simulink model "BuckyWagon_01"  (Simulink 7.7)
settings: Solver=FixedStepDiscrete  StartTime=0.0  StopTime=10.0  RelTol=1e-3
PreLoadFcn:
  | try, eval([bdroot '_setup']); catch, eval('model_setup', ''); end
InitFcn:
  | try, eval([bdroot '_setup']); catch, eval('model_setup', ''); end
undefined symbols (not defined in the file or in its folder): ECU565, High, Low, miniviewSetup, motohawk_build_version, motohawk_get_faults, motohawk_setup_toolchains, motohawk_trunc_name, motohawk_vardec_config_group, motohawk_vardec_path, tc, True
libraries: MotoHawk_lib x594, simulink x27, motohawk_control_primitives_lib x19, miniview_lib x10, MotoHawk_VDOGauge_lib x8, motohawk_engine_lib x5, motohawk_annotations_lib x1
(part 5 of 10)

== system BuckyWagon_01/Foreground/Control Strategy/HV Controller ==
  Battery Ready : Inport
  Contactor Status : Inport  Port=2
  Eaton  Present : Inport  Port=3
  Drive Ready : Inport  Port=4
  Charge Contactor : Inport  Port=5
  Battery has passed power-on-self-test and is ready : simulink/Logic and Bit Operations/Compare To Constant  SystemSampleTime=-1  relop===  const=1  LogicOutDataTypeMode=boolean
  Contacter Controller : Subsystem
  Logical Operator{,1,3..4} (4 alike) : Logic  AllPortsSameDT=off  OutDataTypeStr=boolean
  Logical Operator12 : Logic  Operator=OR  AllPortsSameDT=off  OutDataTypeStr=boolean
  Logical Operator2 : Logic  Operator=NOT  AllPortsSameDT=off  OutDataTypeStr=boolean
  Logical Operator5 : Logic  Operator=OR  AllPortsSameDT=off  OutDataTypeStr=boolean
  Main contactors closed and ready : simulink/Logic and Bit Operations/Compare To Constant  SystemSampleTime=-1  relop===  const=1  LogicOutDataTypeMode=boolean
  motohawk_calibration8 : MotoHawk_lib/Calibration & Probing Blocks/motohawk_calibration  nam='Allow_MainContactor_Close'  val=16  storage=Calibration  show_more=on  name_source=Use Parameter  data_type=boolean  read_level=1  write_level=1  ovr_cals=on  view_as=Number  enum_struct={'Disabled', 'Enabled'}  vector_style=Wide Row  use_help_units=on  help='1=normal mode, 0=prevent main contactors from closing'  units='flag'  use_header_enum=off  row_header_enum={}  col_header_enum={}  use_min_max=on  min_val=0  max_val=1  use_precision=off  precision=''  gain=1  offset=0  exp=1  use_mototune_group=on  mototune_group='Actuators | BCM'
  motohawk_data_def2 : MotoHawk_lib/Data Storage Blocks/motohawk_data_def  nam='Batt_Load_Enable'  container_nam=''  data=0  typ=boolean  struct_nam='MyStruct'  storage=Volatile  outputRef=off  use_vardec=on  window=Display  read_level=1  write_level=1  ovr_cals=on  view_as=Number  enum_struct={'Disabled', 'Enabled'}  vector_style=Wide Row  use_help_units=off  help=''  units=''  use_header_enum=off  row_header_enum=''  col_header_enum=''  use_min_max=off  min_val=-inf  max_val=inf  use_precision=off  precision=''  gain=1  offset=0  exp=1  use_mototune_group=off  mototune_group=motohawk_vardec_path(gcb)  eval_name=MyData  data_stores=motohawk_sfun_data_def_data_stores  struct_instances=motohawk_sfun_data_def_struct_instances  vardecs=motohawk_sfun_data_def_vardecs
  motohawk_data_read : MotoHawk_lib/Data Storage Blocks/motohawk_data_read  source=Lookup By Name  structure=Scalar  operation=Read scalar from location by index  sz_vec=4  sz_row=2  sz_col=3  typ=boolean  nam='Shutdown_Req'  checkNull=on  struct_inst_name='Struct1'  struct_nam='MyStruct'
  motohawk_data_write : MotoHawk_lib/Data Storage Blocks/motohawk_data_write  source=Lookup By Name  structure=Scalar  operation=Write entire data structure at once  sz_vec=9  sz_row=2  sz_col=9  typ=boolean  nam='Batt_Load_Enable'  checkNull=on  write_read_only=off  struct_inst_name=''  struct_name='MyStruct'
  motohawk_fault_action : MotoHawk_lib/Fault Management Blocks/motohawk_fault_action  nam='OpenContactors'  output_status=on  eval_nam=OpenContactors
  motohawk_override_abs2 : MotoHawk_lib/Calibration & Probing Blocks/motohawk_override_abs  SystemSampleTime=-1  parent_name='Contactor_Shutdown_Test'  parent_val=0  show_more=on  name_source=Use Parameter  parent_read_level=1  parent_override_level=1  view_as=Number  enum_struct={'Disabled', 'Enabled'}  use_help_units=off  parent_help=''  parent_units=''  use_min_max=on  parent_min=0  parent_max=1  use_precision=off  parent_precision=''  parent_gain=1  parent_offset=0  parent_exp=1  use_mototune_group=on  parent_group='BuckyWagon_01 | Strategy | Control Strategy | HV Controller'
  Contactor Command : Outport
  DC DC Enable : Outport  Port=2
  Drive Enable : Outport  Port=3
  HV Hydraulic Pump Enable : Outport  Port=4
  wires:
  Battery Ready/1 -> Battery has passed power-on-self-test and is ready/1
  Contactor Status/1 -> Main contactors closed and ready/1
  Battery has passed power-on-self-test and is ready/1 -> Contacter Controller/1(Battery OK)
  Main contactors closed and ready/1 -> Contacter Controller/3(Contactor Status)
  Contacter Controller/1(Contactor Enable) -> Logical Operator/2
  Logical Operator/1 -> Contactor Command/1
  motohawk_calibration8/1 -> Logical Operator/1
  Logical Operator12/1 -> Contacter Controller/2(Shutdown Command)
  motohawk_override_abs2/1 -> Logical Operator12/1
  motohawk_fault_action/1 -> Logical Operator12/2
  Eaton  Present/1 -> Logical Operator2/1
  motohawk_data_read/1 -> Logical Operator1/1
  Logical Operator1/1 -> motohawk_override_abs2/1
  Logical Operator2/1 -> Logical Operator1/2, Logical Operator3/2
  Contacter Controller/2(Load Enable) -> Logical Operator3/1, motohawk_data_write/1, Logical Operator5/1
  Logical Operator3/1 -> Logical Operator4/2, HV Hydraulic Pump Enable/1
  Logical Operator4/1 -> Drive Enable/1
  Drive Ready/1 -> Logical Operator4/1
  Logical Operator5/1 -> DC DC Enable/1
  Charge Contactor/1 -> Logical Operator5/2

== system BuckyWagon_01/Foreground/Control Strategy/Reverse ==
  Inputs : Inport
  Abs : Abs
  Bus Selector2 : BusSelector  OutputSignals=Accel,VehicleSpeed,ReverseSw
  Chart : Stateflow chart  TreatAsAtomicUnit=on
  Constant : Constant
  Switch : Switch  Criteria=u2 ~= 0
  motohawk_calibration : MotoHawk_lib/Calibration & Probing Blocks/motohawk_calibration  nam='fwdAccThres'  val=0.02  storage=Calibration  show_more=on  name_source=Use Parameter  data_type=Inherit from 'Default Value'  read_level=1  write_level=1  ovr_cals=on  view_as=Number  enum_struct={'Disabled', 'Enabled'}  vector_style=Wide Row  use_help_units=on  help='Accelerator must be below this to switch Rev->Fwd'  units='%'  use_header_enum=off  row_header_enum={}  col_header_enum={}  use_min_max=on  min_val=0  max_val=1  use_precision=off  precision=''  gain=1  offset=0  exp=1  use_mototune_group=off  mototune_group=motohawk_vardec_path(gcb)
  motohawk_calibration1 : MotoHawk_lib/Calibration & Probing Blocks/motohawk_calibration  nam='ReverseDerate'  val=-0.6  storage=Calibration  show_more=on  name_source=Use Parameter  data_type=Inherit from 'Default Value'  read_level=1  write_level=1  ovr_cals=on  view_as=Number  enum_struct={'Disabled', 'Enabled'}  vector_style=Wide Row  use_help_units=on  help='Torque Derating Factor in reverse'  units='%'  use_header_enum=off  row_header_enum={}  col_header_enum={}  use_min_max=on  min_val=-1  max_val=0  use_precision=off  precision=''  gain=1  offset=0  exp=1  use_mototune_group=off  mototune_group=motohawk_vardec_path(gcb)
  motohawk_calibration2 : MotoHawk_lib/Calibration & Probing Blocks/motohawk_calibration  nam='fwdSpdThres'  val=5  storage=Calibration  show_more=on  name_source=Use Parameter  data_type=Inherit from 'Default Value'  read_level=1  write_level=1  ovr_cals=on  view_as=Number  enum_struct={'Disabled', 'Enabled'}  vector_style=Wide Row  use_help_units=on  help='Must be below this speed to switch Rev->Fwd'  units='mph'  use_header_enum=off  row_header_enum={}  col_header_enum={}  use_min_max=on  min_val=0  max_val=inf  use_precision=off  precision=''  gain=1  offset=0  exp=1  use_mototune_group=off  mototune_group=motohawk_vardec_path(gcb)
  motohawk_calibration3 : MotoHawk_lib/Calibration & Probing Blocks/motohawk_calibration  nam='offTime'  val=20  storage=Calibration  show_more=on  name_source=Use Parameter  data_type=Inherit from 'Default Value'  read_level=1  write_level=1  ovr_cals=on  view_as=Number  enum_struct={'Disabled', 'Enabled'}  vector_style=Wide Row  use_help_units=on  help='Switch must be released this long to press again.'  units='%'  use_header_enum=off  row_header_enum={}  col_header_enum={}  use_min_max=on  min_val=0  max_val=inf  use_precision=on  precision='1.3'  gain=0.005  offset=0  exp=1  use_mototune_group=on  mototune_group=motohawk_vardec_path(gcb)
  motohawk_calibration4 : MotoHawk_lib/Calibration & Probing Blocks/motohawk_calibration  nam='revAccThres'  val=0.02  storage=Calibration  show_more=on  name_source=Use Parameter  data_type=Inherit from 'Default Value'  read_level=1  write_level=1  ovr_cals=on  view_as=Number  enum_struct={'Disabled', 'Enabled'}  vector_style=Wide Row  use_help_units=on  help='Accelerator must be below this to switch Fwd->Rev'  units='%'  use_header_enum=off  row_header_enum={}  col_header_enum={}  use_min_max=on  min_val=0  max_val=1  use_precision=off  precision=''  gain=1  offset=0  exp=1  use_mototune_group=off  mototune_group=motohawk_vardec_path(gcb)
  motohawk_calibration5 : MotoHawk_lib/Calibration & Probing Blocks/motohawk_calibration  nam='revSpdThres'  val=5  storage=Calibration  show_more=on  name_source=Use Parameter  data_type=Inherit from 'Default Value'  read_level=1  write_level=1  ovr_cals=on  view_as=Number  enum_struct={'Disabled', 'Enabled'}  vector_style=Wide Row  use_help_units=on  help='Must be below this speed to switch Fwd->Rev.'  units='mph'  use_header_enum=off  row_header_enum={}  col_header_enum={}  use_min_max=on  min_val=0  max_val=inf  use_precision=off  precision=''  gain=1  offset=0  exp=1  use_mototune_group=off  mototune_group=motohawk_vardec_path(gcb)
  motohawk_calibration6 : MotoHawk_lib/Calibration & Probing Blocks/motohawk_calibration  nam='onTime'  val=10  storage=Calibration  show_more=on  name_source=Use Parameter  data_type=Inherit from 'Default Value'  read_level=1  write_level=1  ovr_cals=on  view_as=Number  enum_struct={'Disabled', 'Enabled'}  vector_style=Wide Row  use_help_units=on  help='Switch must be pressed this long.'  units='%'  use_header_enum=off  row_header_enum={}  col_header_enum={}  use_min_max=on  min_val=0  max_val=inf  use_precision=on  precision='1.3'  gain=0.005  offset=0  exp=1  use_mototune_group=off  mototune_group=motohawk_vardec_path(gcb)
  motohawk_override_abs : MotoHawk_lib/Calibration & Probing Blocks/motohawk_override_abs  SystemSampleTime=-1  parent_name='In_Reverse'  parent_val=0  show_more=off  name_source=Use Parameter  parent_read_level=1  parent_override_level=1  view_as=Number  enum_struct={'Disabled', 'Enabled'}  use_help_units=off  parent_help=''  parent_units=''  use_min_max=off  parent_min=-inf  parent_max=inf  use_precision=off  parent_precision=''  parent_gain=1  parent_offset=0  parent_exp=1  use_mototune_group=off  parent_group=motohawk_vardec_path(gcb)
  motohawk_probe : MotoHawk_lib/Calibration & Probing Blocks/motohawk_probe  nam='In_Reverse'  show_more=off  name_source=Use Parameter  read_level=1  view_as=Number  enum_struct={'Disabled', 'Enabled'}  vector_style=Wide Row  use_help_units=off  help=''  units=''  use_header_enum=off  row_header_enum={}  col_header_enum={}  use_precision=off  precision=''  gain=1  offset=0  exp=1  use_mototune_group=off  mototune_group=motohawk_vardec_path(gcb)
  InReverse : Outport
  ReverseMult : Outport  Port=2
  wires:
  Inputs/1 -> Bus Selector2/1
  Chart/1(inReverse) -> motohawk_override_abs/1
  motohawk_override_abs/1 -> Switch/2, motohawk_probe/1, InReverse/1
  motohawk_calibration1/1 -> Switch/1
  Constant/1 -> Switch/3
  Switch/1 -> ReverseMult/1
  motohawk_calibration/1 -> Chart/4(fwdAccThres)
  motohawk_calibration2/1 -> Chart/5(fwdSpdThres)
  Bus Selector2/1 -> Chart/1(accel)  "<Accel>"
  Bus Selector2/2 -> Abs/1  "<VehicleSpeed>"
  Bus Selector2/3 -> Chart/3(revButton)  "<ReverseSw>"
  motohawk_calibration4/1 -> Chart/7(revAccThres)
  motohawk_calibration3/1 -> Chart/6(offTime)
  motohawk_calibration5/1 -> Chart/8(revSpdThres)
  motohawk_calibration6/1 -> Chart/9(onTime)
  Abs/1 -> Chart/2(speed)

== system BuckyWagon_01/Foreground/MiniViewDisplay/Down Button ==
  CAN Receive Slot Trigger : MotoHawk_lib/CAN Blocks/CAN Receive Slot Trigger  Tag=Trigger  slot='miniview_button_down'  inherited=on  function_name=Trigger_CAN_Slot_miniview_button_down_2150p0001
  Demux : Demux  Outputs=2
  Subsystem : Subsystem
  Update : Outport
  Down Asserted : Outport  Port=2
  Down Count : Outport  Port=3
  wires:
  Subsystem/2(Out2) -> Down Count/1
  Demux/2 -> Update/1
  CAN Receive Slot Trigger/1 -> Demux/1
  Demux/1 -> Subsystem/Trigger
  Subsystem/1(Out1) -> Down Asserted/1

== system BuckyWagon_01/Foreground/MiniViewDisplay/Enabled Subsystem ==
  In : Inport
  Enable : EnablePort
  Out : Outport
  wires:
  In/1 -> Out/1

== system BuckyWagon_01/Foreground/MiniViewDisplay/Enabled Subsystem1 ==
  In : Inport
  Enable : EnablePort
  Out : Outport
  wires:
  In/1 -> Out/1

== system BuckyWagon_01/Foreground/MiniViewDisplay/Enabled Subsystem2 ==
  In : Inport
  Enable : EnablePort
  Out : Outport
  wires:
  In/1 -> Out/1

== system BuckyWagon_01/Foreground/MiniViewDisplay/Function-Call Subsystem ==
  Value : Inport
  function : TriggerPort  TriggerType=function-call
  motohawk_data_write : MotoHawk_lib/Data Storage Blocks/motohawk_data_write  source=Lookup By Name  structure=Scalar  operation=Write scalar into location by index  sz_vec=-1  sz_row=3  sz_col=2  typ=uint8  nam='listIndex'  checkNull=on  write_read_only=off  struct_inst_name='Struct1'  struct_name='MyStruct'
  wires:
  Value/1 -> motohawk_data_write/1

== system BuckyWagon_01/Foreground/MiniViewDisplay/Function-Call Subsystem1 ==
  Value : Inport
  function : TriggerPort  TriggerType=function-call
  motohawk_data_write : MotoHawk_lib/Data Storage Blocks/motohawk_data_write  source=Lookup By Name  structure=Scalar  operation=Write scalar into location by index  sz_vec=-1  sz_row=3  sz_col=2  typ=uint8  nam='screen'  checkNull=on  write_read_only=off  struct_inst_name='Struct1'  struct_name='MyStruct'
  wires:
  Value/1 -> motohawk_data_write/1

== system BuckyWagon_01/Foreground/MiniViewDisplay/Function-Call Subsystem2 ==
  Value : Inport
  function : TriggerPort  TriggerType=function-call
  motohawk_data_write : MotoHawk_lib/Data Storage Blocks/motohawk_data_write  source=Lookup By Name  structure=Scalar  operation=Write scalar into location by index  sz_vec=-1  sz_row=3  sz_col=2  typ=uint8  nam='singleIndex'  checkNull=on  write_read_only=off  struct_inst_name='Struct1'  struct_name='MyStruct'
  wires:
  Value/1 -> motohawk_data_write/1

== system BuckyWagon_01/Foreground/MiniViewDisplay/Function-Call Subsystem3 ==
  Value : Inport
  function : TriggerPort  TriggerType=function-call
  motohawk_data_write : MotoHawk_lib/Data Storage Blocks/motohawk_data_write  source=Lookup By Name  structure=Vector  operation=Write entire data structure at once  sz_vec=2  sz_row=3  sz_col=2  typ=uint8  nam='dualIndex'  checkNull=on  write_read_only=off  struct_inst_name='Struct1'  struct_name='MyStruct'
  wires:
  Value/1 -> motohawk_data_write/1

== system BuckyWagon_01/Foreground/MiniViewDisplay/Function-Call Subsystem4 ==
  Value : Inport
  function : TriggerPort  TriggerType=function-call
  motohawk_data_write : MotoHawk_lib/Data Storage Blocks/motohawk_data_write  source=Lookup By Name  structure=Vector  operation=Write entire data structure at once  sz_vec=4  sz_row=3  sz_col=2  typ=uint8  nam='quadIndex'  checkNull=on  write_read_only=off  struct_inst_name='Struct1'  struct_name='MyStruct'
  wires:
  Value/1 -> motohawk_data_write/1

== system BuckyWagon_01/Foreground/MiniViewDisplay/GetFaultName ==
  Chart : Stateflow chart  TreatAsAtomicUnit=on
  Fault Iterator : Subsystem  TreatAsAtomicUnit=on
  Unit Delay : UnitDelay  SampleTime=-1
  Unit Delay1 : UnitDelay  SampleTime=-1
  getStringLength : Stateflow chart  TreatAsAtomicUnit=on
  motohawk_calibration : MotoHawk_lib/Calibration & Probing Blocks/motohawk_calibration  nam='DisplayFaults'  val=1  storage=Calibration  show_more=on  name_source=Use Parameter  data_type=boolean  read_level=1  write_level=1  ovr_cals=on  view_as=Enumeration  enum_struct={'Disabled', 'Enabled'}  vector_style=Wide Row  use_help_units=on  help='Enable displaying faults when they are active.'  units=''  use_header_enum=off  row_header_enum={}  col_header_enum={}  use_min_max=off  min_val=-inf  max_val=inf  use_precision=off  precision=''  gain=1  offset=0  exp=1  use_mototune_group=off  mototune_group=motohawk_vardec_path(gcb)
  motohawk_calibration1 : MotoHawk_lib/Calibration & Probing Blocks/motohawk_calibration  nam='InvertMode'  val=0  storage=Calibration  show_more=on  name_source=Use Parameter  data_type=boolean  read_level=1  write_level=1  ovr_cals=on  view_as=Enumeration  enum_struct={'Normal', 'Inverted'}  vector_style=Wide Row  use_help_units=on  help='Sets the background color for the text.'  units=''  use_header_enum=off  row_header_enum={}  col_header_enum={}  use_min_max=off  min_val=-inf  max_val=inf  use_precision=off  precision=''  gain=1  offset=0  exp=1  use_mototune_group=off  mototune_group=motohawk_vardec_path(gcb)
  motohawk_calibration2 : MotoHawk_lib/Calibration & Probing Blocks/motohawk_calibration  nam='noErrText'  val=uint8([32 66 117 99 107 69 86 0 0 0])  storage=Calibration  show_more=on  name_source=Use Parameter  data_type=uint8  read_level=1  write_level=1  ovr_cals=on  view_as=Text  enum_struct={'Disabled', 'Enabled'}  vector_style=Wide Row  use_help_units=on  help='Text to display if there are no faults.'  units=''  use_header_enum=off  row_header_enum={}  col_header_enum={}  use_min_max=off  min_val=-inf  max_val=inf  use_precision=off  precision=''  gain=1  offset=0  exp=1  use_mototune_group=off  mototune_group=motohawk_vardec_path(gcb)
  motohawk_calibration3 : MotoHawk_lib/Calibration & Probing Blocks/motohawk_calibration  nam='dispLength'  val=6  storage=Calibration  show_more=on  name_source=Use Parameter  data_type=uint8  read_level=1  write_level=1  ovr_cals=on  view_as=Number  enum_struct={'Disabled', 'Enabled'}  vector_style=Wide Row  use_help_units=on  help='Number of characters to display when scrolling fault name.'  units=''  use_header_enum=off  row_header_enum={}  col_header_enum={}  use_min_max=on  min_val=0  max_val=9  use_precision=on  precision=''  gain=1  offset=0  exp=1  use_mototune_group=off  mototune_group=motohawk_vardec_path(gcb)
  motohawk_calibration4 : MotoHawk_lib/Calibration & Probing Blocks/motohawk_calibration  nam='lastScrollTime'  val=100  storage=Calibration  show_more=on  name_source=Use Parameter  data_type=uint16  read_level=1  write_level=1  ovr_cals=on  view_as=Number  enum_struct={'Disabled', 'Enabled'}  vector_style=Wide Row  use_help_units=on  help='Time to spend on the last view of the scroll'  units='s'  use_header_enum=off  row_header_enum={}  col_header_enum={}  use_min_max=on  min_val=0  max_val=5  use_precision=on  precision='1.3'  gain=0.005  offset=0  exp=1  use_mototune_group=off  mototune_group=motohawk_vardec_path(gcb)
  motohawk_calibration5 : MotoHawk_lib/Calibration & Probing Blocks/motohawk_calibration  nam='scrollTime'  val=40  storage=Calibration  show_more=on  name_source=Use Parameter  data_type=uint16  read_level=1  write_level=1  ovr_cals=on  view_as=Number  enum_struct={'Disabled', 'Enabled'}  vector_style=Wide Row  use_help_units=on  help='Time to spend on each view of the scroll'  units='s'  use_header_enum=off  row_header_enum={}  col_header_enum={}  use_min_max=on  min_val=0  max_val=5  use_precision=on  precision='1.3'  gain=0.005  offset=0  exp=1  use_mototune_group=off  mototune_group=motohawk_vardec_path(gcb)
  motohawk_calibration6 : MotoHawk_lib/Calibration & Probing Blocks/motohawk_calibration  nam='minTime'  val=300  storage=Calibration  show_more=on  name_source=Use Parameter  data_type=uint16  read_level=1  write_level=1  ovr_cals=on  view_as=Number  enum_struct={'Disabled', 'Enabled'}  vector_style=Wide Row  use_help_units=on  help='Minimum time to display each fault name.'  units='s'  use_header_enum=off  row_header_enum={}  col_header_enum={}  use_min_max=on  min_val=0  max_val=5  use_precision=on  precision='1.3'  gain=0.005  offset=0  exp=1  use_mototune_group=off  mototune_group=motohawk_vardec_path(gcb)
  motohawk_calibration7 : MotoHawk_lib/Calibration & Probing Blocks/motohawk_calibration  nam='firstScrollTime'  val=200  storage=Calibration  show_more=on  name_source=Use Parameter  data_type=uint16  read_level=1  write_level=1  ovr_cals=on  view_as=Number  enum_struct={'Disabled', 'Enabled'}  vector_style=Wide Row  use_help_units=on  help='Time to spend on first view of the scroll'  units='s'  use_header_enum=off  row_header_enum={}  col_header_enum={}  use_min_max=on  min_val=0  max_val=5  use_precision=on  precision='1.3'  gain=0.005  offset=0  exp=1  use_mototune_group=off  mototune_group=motohawk_vardec_path(gcb)
  motohawk_probe : MotoHawk_lib/Calibration & Probing Blocks/motohawk_probe  nam='minTimer'  show_more=on  name_source=Use Parameter  read_level=1  view_as=Number  enum_struct={'Disabled', 'Enabled'}  vector_style=Wide Row  use_help_units=off  help=''  units=''  use_header_enum=off  row_header_enum={}  col_header_enum={}  use_precision=on  precision='1.3'  gain=0.005  offset=0  exp=1  use_mototune_group=off  mototune_group=motohawk_vardec_path(gcb)
  motohawk_probe2 : MotoHawk_lib/Calibration & Probing Blocks/motohawk_probe  nam='scrollTimer'  show_more=on  name_source=Use Parameter  read_level=1  view_as=Number  enum_struct={'Disabled', 'Enabled'}  vector_style=Wide Row  use_help_units=off  help=''  units=''  use_header_enum=off  row_header_enum={}  col_header_enum={}  use_precision=on  precision='1.3'  gain=0.005  offset=0  exp=1  use_mototune_group=off  mototune_group=motohawk_vardec_path(gcb)
  motohawk_probe3 : MotoHawk_lib/Calibration & Probing Blocks/motohawk_probe  nam='scrollIndex'  show_more=off  name_source=Use Parameter  read_level=1  view_as=Number  enum_struct={'Disabled', 'Enabled'}  vector_style=Wide Row  use_help_units=off  help=''  units=''  use_header_enum=off  row_header_enum={}  col_header_enum={}  use_precision=off  precision=''  gain=1  offset=0  exp=1  use_mototune_group=off  mototune_group=motohawk_vardec_path(gcb)
  Name : Outport
  Mode : Outport  Port=2
  wires:
  Chart/6(getNewFault) -> Fault Iterator/Trigger
  Chart/2(text) -> Name/1
  Chart/1(mode) -> Mode/1
  Chart/3(minTimer) -> motohawk_probe/1
  Chart/4(scrollIndex) -> motohawk_probe3/1
  Chart/5(scrollTimer) -> motohawk_probe2/1
  motohawk_calibration/1 -> Chart/7(dispFaults)
  motohawk_calibration1/1 -> Chart/1(invertMode)
  motohawk_calibration2/1 -> Chart/2(noErrText)
  motohawk_calibration3/1 -> Chart/3(dispLength)
  Fault Iterator/2(valid) -> Unit Delay1/1
  Fault Iterator/1(Name) -> Unit Delay/1
  motohawk_calibration4/1 -> Chart/4(lastScrollTime)
  motohawk_calibration5/1 -> Chart/5(scrollTime)
  motohawk_calibration6/1 -> Chart/8(minTime)
  getStringLength/1(faultNameLength) -> Chart/9(faultNameLen)
  Unit Delay/1 -> Chart/10(faultName), getStringLength/1(faultName)
  Unit Delay1/1 -> Chart/11(faultValid)
  motohawk_calibration7/1 -> Chart/6(firstScrollTime)

== system BuckyWagon_01/Foreground/MiniViewDisplay/Menu Button ==
  CAN Receive Slot Trigger : MotoHawk_lib/CAN Blocks/CAN Receive Slot Trigger  Tag=Trigger  slot='miniview_button_menu'  inherited=on  function_name=Trigger_CAN_Slot_miniview_button_menu_2408p0001
  Demux : Demux  Outputs=2
  Subsystem : Subsystem
  Update : Outport
  Menu Asserted : Outport  Port=2
  Menu Count : Outport  Port=3
  wires:
  Subsystem/1(Out1) -> Menu Asserted/1
  Demux/1 -> Subsystem/Trigger
  CAN Receive Slot Trigger/1 -> Demux/1
  Demux/2 -> Update/1
  Subsystem/2(Out2) -> Menu Count/1

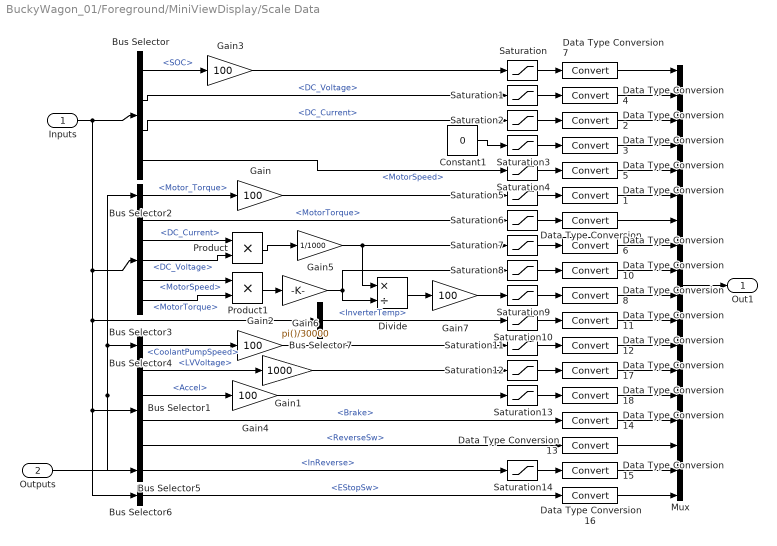
== system BuckyWagon_01/Foreground/MiniViewDisplay/Scale Data ==
  Inputs : Inport
  Outputs : Inport  Port=2
  Bus Selector : BusSelector  OutputSignals=SOC,DC_Voltage,DC_Current,MotorSpeed
  Bus Selector1 : BusSelector  OutputSignals=LVVoltage,Accel,Brake,ReverseSw
  Bus Selector2 : BusSelector  OutputSignals=Motor_Torque
  Bus Selector3 : BusSelector  OutputSignals=MotorTorque,DC_Current,DC_Voltage,MotorSpeed,MotorTorque
  Bus Selector4 : BusSelector  OutputSignals=CoolantPumpSpeed
  Bus Selector5 : BusSelector  OutputSignals=InReverse
  Bus Selector6 : BusSelector  OutputSignals=EStopSw
  Bus Selector7 : BusSelector  OutputSignals=InverterTemp
  Constant1 : Constant  Value=0
  Data Type Conversion{,1..8,10..18} (18 alike) : DataTypeConversion
  Divide : Product  Inputs=*/
  Gain{,2..4,7} (5 alike) : Gain  Gain=100  OutDataTypeStr=Inherit: Inherit via back propagation
  Gain1 : Gain  Gain=1000  OutDataTypeStr=Inherit: Inherit via back propagation
  Gain5 : Gain  Gain=1/1000  OutDataTypeStr=Inherit: Inherit via back propagation
  Gain6 : Gain  Gain=pi()/30000  OutDataTypeStr=Inherit: Inherit via back propagation
  Mux : Mux  Inputs=18
  Product : Product  RndMeth=Zero
  Product1 : Product  RndMeth=Zero
  Saturation{,1..8,10..14} (14 alike) : Saturate  UpperLimit=32767  LowerLimit=-32767
  Saturation9 : Saturate  UpperLimit=100  LowerLimit=0
  Out1 : Outport
  wires:
  Outputs/1 -> Bus Selector2/1, Bus Selector4/1, Bus Selector5/1
  Bus Selector/3 -> Saturation2/1  "<DC_Current>"
  Bus Selector/2 -> Saturation1/1  "<DC_Voltage>"
  Bus Selector/1 -> Gain3/1  "<SOC>"
  Mux/1 -> Out1/1
  Gain3/1 -> Saturation/1
  Data Type Conversion4/1 -> Mux/2
  Data Type Conversion2/1 -> Mux/3
  Data Type Conversion3/1 -> Mux/4
  Data Type Conversion5/1 -> Mux/5
  Gain/1 -> Saturation5/1
  Bus Selector2/1 -> Gain/1  "<Motor_Torque>"
  Inputs/1 -> Bus Selector/1, Bus Selector3/1, Bus Selector1/1, Bus Selector6/1, Bus Selector7/1
  Bus Selector3/1 -> Saturation6/1  "<MotorTorque>"
  Bus Selector3/2 -> Product/1  "<DC_Current>"
  Bus Selector3/3 -> Product/2  "<DC_Voltage>"
  Product/1 -> Gain5/1
  Bus Selector3/4 -> Product1/1  "<MotorSpeed>"
  Bus Selector3/5 -> Product1/2  "<MotorTorque>"
  Product1/1 -> Gain6/1
  Bus Selector7/1 -> Saturation10/1  "<InverterTemp>"
  Gain5/1 -> Divide/1, Saturation7/1
  Gain6/1 -> Divide/2, Saturation8/1
  Data Type Conversion/1 -> Mux/7
  Divide/1 -> Gain7/1
  Gain7/1 -> Saturation9/1
  Data Type Conversion6/1 -> Mux/8
  Data Type Conversion10/1 -> Mux/9
  Bus Selector4/1 -> Gain2/1  "<CoolantPumpSpeed>"
  Gain2/1 -> Saturation11/1
  Bus Selector1/1 -> Gain1/1  "<LVVoltage>"
  Bus Selector1/2 -> Gain4/1  "<Accel>"
  Bus Selector1/3 -> Data Type Conversion14/1  "<Brake>"
  Bus Selector1/4 -> Data Type Conversion13/1  "<ReverseSw>"
  Gain1/1 -> Saturation12/1
  Gain4/1 -> Saturation13/1
  Data Type Conversion14/1 -> Mux/15
  Data Type Conversion13/1 -> Mux/16
  Bus Selector5/1 -> Saturation14/1  "<InReverse>"
  Data Type Conversion15/1 -> Mux/17
  Bus Selector6/1 -> Data Type Conversion16/1  "<EStopSw>"
  Data Type Conversion16/1 -> Mux/18
  Data Type Conversion1/1 -> Mux/6
  Data Type Conversion7/1 -> Mux/1
  Data Type Conversion8/1 -> Mux/10
  Data Type Conversion11/1 -> Mux/11
  Data Type Conversion12/1 -> Mux/12
  Data Type Conversion17/1 -> Mux/13
  Data Type Conversion18/1 -> Mux/14
  Saturation/1 -> Data Type Conversion7/1
  Saturation1/1 -> Data Type Conversion4/1
  Saturation2/1 -> Data Type Conversion2/1
  Saturation3/1 -> Data Type Conversion3/1
  Saturation4/1 -> Data Type Conversion5/1
  Saturation5/1 -> Data Type Conversion1/1
  Saturation6/1 -> Data Type Conversion/1
  Saturation7/1 -> Data Type Conversion6/1
  Saturation8/1 -> Data Type Conversion10/1
  Saturation9/1 -> Data Type Conversion8/1
  Saturation10/1 -> Data Type Conversion11/1
  Saturation11/1 -> Data Type Conversion12/1
  Saturation12/1 -> Data Type Conversion17/1
  Saturation13/1 -> Data Type Conversion18/1
  Saturation14/1 -> Data Type Conversion15/1
  Bus Selector/4 -> Saturation4/1  "<MotorSpeed>"
  Constant1/1 -> Saturation3/1

== system BuckyWagon_01/Foreground/MiniViewDisplay/Send String_efficient ==
  string # : Inport
  string : Inport  Port=2
  Trigger : TriggerPort  TriggerType=function-call
  Demux : Demux  Outputs=2
  Function-Call Generator : simulink/Ports & Subsystems/Function-Call Generator  sample_time=-1  numberOfIterations=1
  Signal Specification : SignalSpecification  OutDataTypeStr=uint8  Dimensions=18
  Subsystem : Subsystem
  Next : Outport
  wires:
  Signal Specification/1 -> Subsystem/2(string)
  Demux/2 -> Next/1
  Function-Call Generator/1 -> Demux/1
  Demux/1 -> Subsystem/Trigger
  string/1 -> Signal Specification/1  "b0"
  string #/1 -> Subsystem/1(string #)  "string"

== system BuckyWagon_01/Foreground/MiniViewDisplay/Up Button ==
  CAN Receive Slot Trigger : MotoHawk_lib/CAN Blocks/CAN Receive Slot Trigger  Tag=Trigger  slot='miniview_button_up'  inherited=on  function_name=Trigger_CAN_Slot_miniview_button_up_2659p0004
  Demux : Demux  Outputs=2
  Subsystem : Subsystem
  Update : Outport
  Up Asserted : Outport  Port=2
  Up Count : Outport  Port=3
  wires:
  Subsystem/2(Up Count) -> Up Count/1
  Demux/2 -> Update/1
  CAN Receive Slot Trigger/1 -> Demux/1
  Demux/1 -> Subsystem/Trigger
  Subsystem/1(Up Asserted) -> Up Asserted/1

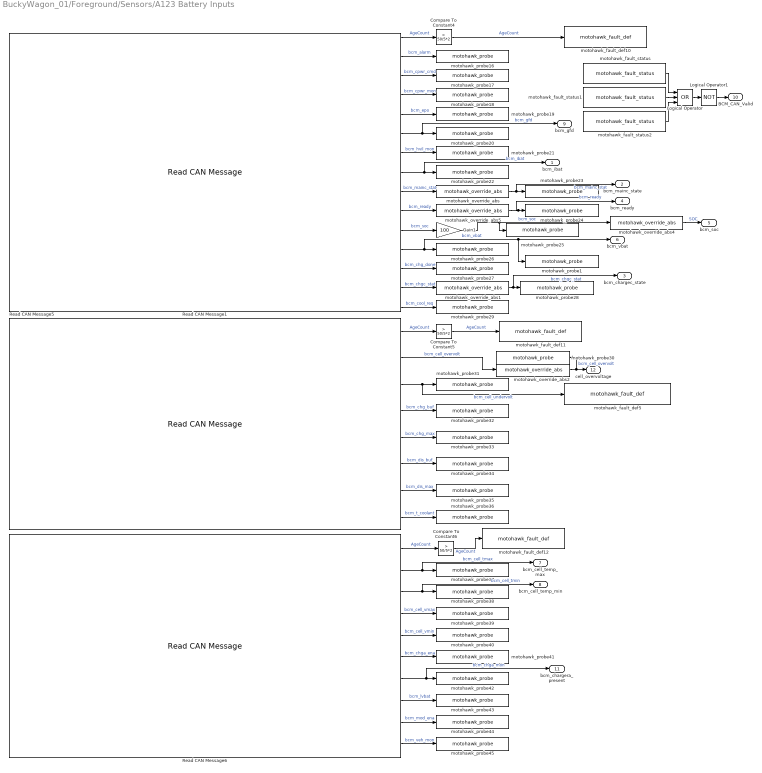
== system BuckyWagon_01/Foreground/Sensors/A123 Battery Inputs ==
  Compare To Constant4 : simulink/Logic and Bit Operations/Compare To Constant  SystemSampleTime=-1  relop=>  const=50/5*2  LogicOutDataTypeMode=boolean  ZeroCross=off
  Compare To Constant5 : simulink/Logic and Bit Operations/Compare To Constant  SystemSampleTime=-1  relop=>  const=50/5*2  LogicOutDataTypeMode=boolean  ZeroCross=off
  Compare To Constant6 : simulink/Logic and Bit Operations/Compare To Constant  SystemSampleTime=-1  relop=>  const=50/5*2  LogicOutDataTypeMode=boolean  ZeroCross=off
  Gain1 : Gain  Gain=100
  Logical Operator : Logic  Operator=OR  Inputs=3  AllPortsSameDT=off  OutDataTypeStr=boolean
  Logical Operator1 : Logic  Operator=NOT  Inputs=3  AllPortsSameDT=off  OutDataTypeStr=boolean
  Read CAN Message1 : MotoHawk_lib/CAN Blocks/Read CAN Message  nam='CAN_2'  bus=-2  msg=BMS_A123_410  queue=1  slot=''  valid=off  stale=on  labelwires=on
  Read CAN Message5 : MotoHawk_lib/CAN Blocks/Read CAN Message  nam='CAN_2'  bus=-2  msg=BMS_A123_420  queue=1  slot=''  valid=off  stale=on  labelwires=on
  Read CAN Message6 : MotoHawk_lib/CAN Blocks/Read CAN Message  nam='CAN_2'  bus=-2  msg=BMS_A123_430  queue=1  slot=''  valid=off  stale=on  labelwires=on
  motohawk_fault_def10 : MotoHawk_lib/Fault Management Blocks/motohawk_fault_def  nam='NoCAN_BCM_410'  mode=Enabled  id=0  x=10  y=20  input_suspected=on  indeterminate=off  increment_xy=on  downsample_count=1  ovr_cals=on  ovr_actions=on  show_actions=off  action1_name=''  action1_cond=(None)  action2_name=''  action2_cond=(None)  action3_name=''  action3_cond=(None)  action4_name=''  action4_cond=(None)
  motohawk_fault_def11 : MotoHawk_lib/Fault Management Blocks/motohawk_fault_def  nam='NoCAN_BCM_420'  mode=Enabled  id=0  x=10  y=20  input_suspected=on  indeterminate=off  increment_xy=on  downsample_count=1  ovr_cals=on  ovr_actions=on  show_actions=off  action1_name=''  action1_cond=(None)  action2_name=''  action2_cond=(None)  action3_name=''  action3_cond=(None)  action4_name=''  action4_cond=(None)
  motohawk_fault_def12 : MotoHawk_lib/Fault Management Blocks/motohawk_fault_def  nam='NoCAN_BCM_430'  mode=Enabled  id=0  x=10  y=20  input_suspected=on  indeterminate=off  increment_xy=on  downsample_count=1  ovr_cals=on  ovr_actions=on  show_actions=off  action1_name=''  action1_cond=(None)  action2_name=''  action2_cond=(None)  action3_name=''  action3_cond=(None)  action4_name=''  action4_cond=(None)
  motohawk_fault_def5 : MotoHawk_lib/Fault Management Blocks/motohawk_fault_def  nam='High_Cell_Voltage_Shutdown'  mode=Sticky  id=[]  x=100  y=200  input_suspected=on  indeterminate=off  increment_xy=on  downsample_count=1  ovr_cals=on  ovr_actions=on  show_actions=on  action1_name='OpenContactors'  action1_cond=Active  action2_name=''  action2_cond=(None)  action3_name=''  action3_cond=(None)  action4_name=''  action4_cond=(None)
  motohawk_fault_status : MotoHawk_lib/Fault Management Blocks/motohawk_fault_status  source=Lookup By Name  nam='NoCAN_BCM_410'  status=Active
  motohawk_fault_status1 : MotoHawk_lib/Fault Management Blocks/motohawk_fault_status  source=Lookup By Name  nam='NoCAN_BCM_420'  status=Active
  motohawk_fault_status2 : MotoHawk_lib/Fault Management Blocks/motohawk_fault_status  source=Lookup By Name  nam='NoCAN_BCM_430'  status=Active
  motohawk_override_abs : MotoHawk_lib/Calibration & Probing Blocks/motohawk_override_abs  SystemSampleTime=-1  parent_name='bcm_mainc_stat'  parent_val=0  show_more=on  name_source=Use Parameter  parent_read_level=1  parent_override_level=1  view_as=Number  enum_struct={'Disabled', 'Enabled'}  use_help_units=off  parent_help=''  parent_units=''  use_min_max=off  parent_min=-inf  parent_max=inf  use_precision=off  parent_precision=''  parent_gain=1  parent_offset=0  parent_exp=1  use_mototune_group=on  parent_group='Sensors | BCM'
  motohawk_override_abs1 : MotoHawk_lib/Calibration & Probing Blocks/motohawk_override_abs  SystemSampleTime=-1  parent_name='bcm_chargec_stat'  parent_val=0  show_more=on  name_source=Use Parameter  parent_read_level=1  parent_override_level=1  view_as=Number  enum_struct={'Disabled', 'Enabled'}  use_help_units=off  parent_help=''  parent_units=''  use_min_max=off  parent_min=-inf  parent_max=inf  use_precision=off  parent_precision=''  parent_gain=1  parent_offset=0  parent_exp=1  use_mototune_group=on  parent_group='Sensors | BCM'
  motohawk_override_abs2 : MotoHawk_lib/Calibration & Probing Blocks/motohawk_override_abs  SystemSampleTime=-1  parent_name='bcm_cell_overvolt_ovr'  parent_val=0  show_more=on  name_source=Use Parameter  parent_read_level=1  parent_override_level=1  view_as=Number  enum_struct={'Disabled', 'Enabled'}  use_help_units=off  parent_help=''  parent_units=''  use_min_max=off  parent_min=-inf  parent_max=inf  use_precision=off  parent_precision=''  parent_gain=1  parent_offset=0  parent_exp=1  use_mototune_group=on  parent_group='Sensors | BCM'
  motohawk_override_abs4 : MotoHawk_lib/Calibration & Probing Blocks/motohawk_override_abs  SystemSampleTime=-1  parent_name='SOC'  parent_val=0.5  show_more=on  name_source=Use Parameter  parent_read_level=1  parent_override_level=1  view_as=Number  enum_struct={'Disabled', 'Enabled'}  use_help_units=off  parent_help=''  parent_units=''  use_min_max=on  parent_min=0  parent_max=1  use_precision=off  parent_precision=''  parent_gain=1  parent_offset=0  parent_exp=1  use_mototune_group=on  parent_group='Sensors | BCM'
  motohawk_override_abs5 : MotoHawk_lib/Calibration & Probing Blocks/motohawk_override_abs  SystemSampleTime=-1  parent_name='bcm_ready'  parent_val=0  show_more=on  name_source=Use Parameter  parent_read_level=1  parent_override_level=1  view_as=Number  enum_struct={'Disabled', 'Enabled'}  use_help_units=off  parent_help=''  parent_units=''  use_min_max=off  parent_min=-inf  parent_max=inf  use_precision=off  parent_precision=''  parent_gain=1  parent_offset=0  parent_exp=1  use_mototune_group=on  parent_group='Sensors | BCM'
  motohawk_probe1 : MotoHawk_lib/Calibration & Probing Blocks/motohawk_probe  nam='DC_Voltage'  show_more=on  name_source=Use Parameter  read_level=1  view_as=Number  enum_struct={'Disabled', 'Enabled'}  vector_style=Wide Row  use_help_units=off  help=''  units=''  use_header_enum=off  row_header_enum={}  col_header_enum={}  use_precision=off  precision=''  gain=1  offset=0  exp=1  use_mototune_group=on  mototune_group='Sensors'
  motohawk_probe{16..29,31..45} (29 alike) : MotoHawk_lib/Calibration & Probing Blocks/motohawk_probe  nam='Probe'  show_more=on  name_source=Use Input Wire Name  read_level=1  view_as=Number  enum_struct={'Disabled', 'Enabled'}  vector_style=Wide Row  use_help_units=off  help=''  units=''  use_header_enum=off  row_header_enum={}  col_header_enum={}  use_precision=off  precision=''  gain=1  offset=0  exp=1  use_mototune_group=on  mototune_group='Sensors | BCM'
  motohawk_probe30 : MotoHawk_lib/Calibration & Probing Blocks/motohawk_probe  nam='bcm_cell_overvolt_probe'  show_more=on  name_source=Use Parameter  read_level=1  view_as=Number  enum_struct={'Disabled', 'Enabled'}  vector_style=Wide Row  use_help_units=off  help=''  units=''  use_header_enum=off  row_header_enum={}  col_header_enum={}  use_precision=off  precision=''  gain=1  offset=0  exp=1  use_mototune_group=on  mototune_group='Sensors | BCM'
  bcm_ibat : Outport
  bcm_mainc_state : Outport  Port=2
  bcm_chargec_state : Outport  Port=3
  bcm_ready : Outport  Port=4
  bcm_soc : Outport  Port=5
  bcm_vbat : Outport  Port=6
  bcm_cell_temp_max : Outport  Port=7
  bcm_cell_temp_min : Outport  Port=8
  bcm_gfd : Outport  Port=9
  BCM_CAN_Valid : Outport  Port=10
  bcm_chargera_present : Outport  Port=11
  cell_overvoltage : Outport  Port=12
  wires:
  Read CAN Message1/2 -> motohawk_probe16/1  "bcm_alarm"
  Read CAN Message1/3 -> motohawk_probe17/1  "bcm_cpwr_cmd"
  Read CAN Message1/4 -> motohawk_probe18/1  "bcm_cpwr_mon"
  Read CAN Message1/5 -> motohawk_probe19/1  "bcm_epo"
  Read CAN Message1/6 -> motohawk_probe20/1, bcm_gfd/1  "bcm_gfd"
  Read CAN Message1/7 -> motohawk_probe21/1  "bcm_hvil_mon"
  Read CAN Message1/8 -> motohawk_probe22/1, bcm_ibat/1  "bcm_ibat"
  Read CAN Message1/9 -> motohawk_override_abs/1  "bcm_mainc_stat"
  Read CAN Message1/10 -> motohawk_override_abs5/1  "bcm_ready"
  Read CAN Message1/11 -> Gain1/1  "bcm_soc"
  Read CAN Message1/12 -> motohawk_probe26/1, motohawk_probe1/1, bcm_vbat/1  "bcm_vbat"
  Read CAN Message1/13 -> motohawk_probe27/1  "bcm_chg_done"
  Read CAN Message1/14 -> motohawk_override_abs1/1  "bcm_chgc_stat"
  Read CAN Message1/15 -> motohawk_probe29/1  "bcm_cool_req"
  Read CAN Message5/2 -> motohawk_override_abs2/1  "bcm_cell_overvolt"
  Read CAN Message5/3 -> motohawk_probe31/1, motohawk_fault_def5/1  "bcm_cell_undervolt"
  Read CAN Message5/4 -> motohawk_probe32/1  "bcm_chg_buf"
  Read CAN Message5/5 -> motohawk_probe33/1  "bcm_chg_max"
  Read CAN Message5/6 -> motohawk_probe34/1  "bcm_dis_buf"
  Read CAN Message5/7 -> motohawk_probe35/1  "bcm_dis_max"
  Read CAN Message5/8 -> motohawk_probe36/1  "bcm_t_coolant"
  Read CAN Message6/2 -> motohawk_probe37/1, bcm_cell_temp_max/1  "bcm_cell_tmax"
  Read CAN Message6/3 -> motohawk_probe38/1, bcm_cell_temp_min/1  "bcm_cell_tmin"
  Read CAN Message6/4 -> motohawk_probe39/1  "bcm_cell_vmax"
  Read CAN Message6/5 -> motohawk_probe40/1  "bcm_cell_vmin"
  Read CAN Message6/6 -> motohawk_probe41/1  "bcm_chga_ena"
  Read CAN Message6/7 -> motohawk_probe42/1, bcm_chargera_present/1  "bcm_chga_mon"
  Read CAN Message6/8 -> motohawk_probe43/1  "bcm_lvbat"
  Read CAN Message6/9 -> motohawk_probe44/1  "bcm_mod_ena"
  Read CAN Message6/10 -> motohawk_probe45/1  "bcm_veh_mon"
  Compare To Constant4/1 -> motohawk_fault_def10/1  "AgeCount"
  Read CAN Message1/1 -> Compare To Constant4/1  "AgeCount"
  Compare To Constant5/1 -> motohawk_fault_def11/1  "AgeCount"
  Read CAN Message5/1 -> Compare To Constant5/1  "AgeCount"
  Compare To Constant6/1 -> motohawk_fault_def12/1  "AgeCount"
  Read CAN Message6/1 -> Compare To Constant6/1  "AgeCount"
  motohawk_override_abs4/1 -> bcm_soc/1  "SOC"
  motohawk_override_abs/1 -> motohawk_probe23/1, bcm_mainc_state/1  "bcm_mainc_stat"
  motohawk_override_abs5/1 -> motohawk_probe24/1, bcm_ready/1  "bcm_ready"
  motohawk_fault_status/1 -> Logical Operator/1
  motohawk_fault_status1/1 -> Logical Operator/2
  motohawk_fault_status2/1 -> Logical Operator/3
  Logical Operator/1 -> Logical Operator1/1
  Logical Operator1/1 -> BCM_CAN_Valid/1
  motohawk_override_abs1/1 -> motohawk_probe28/1, bcm_chargec_state/1  "bcm_chgc_stat"
  Gain1/1 -> motohawk_override_abs4/1, motohawk_probe25/1  "bcm_soc"
  motohawk_override_abs2/1 -> cell_overvoltage/1, motohawk_probe30/1  "bcm_cell_overvolt"
